simulink model "sgMdl_IO3xx_Resolver_Emulation_Setup"  (R2024b)
settings: Solver=FixedStepAuto  StartTime=0.0  StopTime=inf  RelTol=1e-3
undefined symbols (not defined in the file): Ended, Pull, pull, Single, up
libraries: speedgoatlib_fpga_analog_io x1, speedgoatlib_fpga_resolver x1, speedgoatlib_fpga x1
Description:
  | IO3xx Resolver Emulation - Setup
settings Model: ModifiedByFormat=Speedgoat  SimulationMode=external  ExtModeTrigDuration=100000  Creator=Speedgoat  LastModifiedBy=Speedgoat
settings SolverCC: ConcurrentTasks=on  PositivePriorityOrder=on
settings OptimizationCC: BlockReduction=off  OptimizeBlockIOStorage=off  ReuseModelBlockBuffer=off
settings DebuggingCC: TasksWithSamePriorityMsg=none
settings HardwareCC: ProdBitPerLong=64  ProdLongLongMode=on  ProdHWDeviceType=Intel->x86-64 (Linux 64)
settings ModelReferenceCC: EnableRefExpFcnMdlSchedulingChecks=on
settings RTWCC: Description=Speedgoat Real-Time Target Machine  SystemTargetFile=speedgoat.tlc  TemplateMakefile=slrealtime_default_tmf  Toolchain=Simulink Real-Time Toolchain  BuildConfiguration=Faster Runs  TargetLang=C++  GPUComputeCapability=3.5
settings SimulinkRealTimeTargetCC: SubcomponentCodeInterfacePackaging=Reusable function  InstructionSetFMA=off  LogToMDFFile=off  SLRTFileLogMaxRuns=10
settings ConfigComp: CovBoundaryAbsTol=1.0e-5

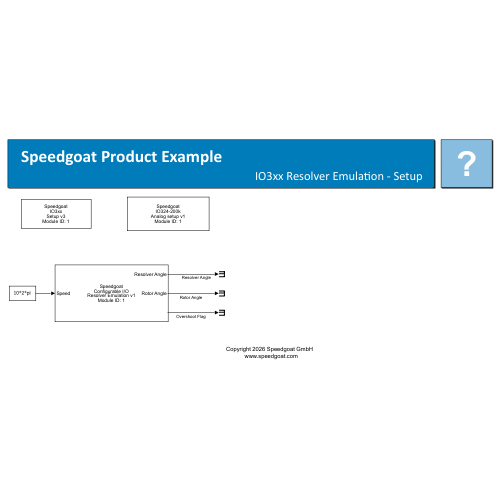
[thumbnail: Simulink's stored preview of the top-level diagram]
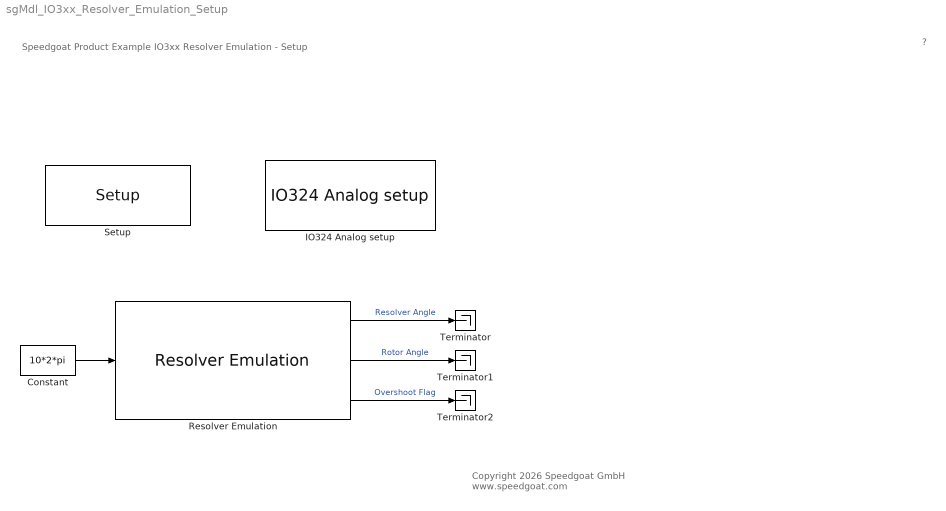
== system sgMdl_IO3xx_Resolver_Emulation_Setup ==
  note: Speedgoat Product Example
      | IO3xx Resolver Emulation - Setup
  note: ?
  note: Copyright 2026 Speedgoat GmbH
      |  www.speedgoat.com
  Constant : Constant  Value=10*2*pi  SampleTime=1e-3
  IO324 Analog setup : speedgoatlib_fpga_analog_io/IO324/IO324 Analog setup  id=1  parEnableCodeModule1=on  parEnableCodeModule2=off  parEnableCodeModule3=off  parEnableCodeModule4=off  parEnableCodeModule5=off  parEnableCodeModule6=off  parEnableCodeModule7=off  parEnableCodeModule8=off  parAdcEnableIndividualTrigger=off  parAdcTriggerMode1=I/O Module Internal Signal  parAdcSampleRate1=100e3  parAdcDioTriggerChannel1=1  parAdcInternalTrigger1=<empty>  parAdcOversampling1=None  parAdcTriggerMode2=Model Step  parAdcSampleRate2=100e3  parAdcDioTriggerChannel2=1  parAdcInternalTrigger2=<empty>  parAdcOversampling2=None  parAdcTriggerMode3=Model Step  parAdcSampleRate3=100e3  parAdcDioTriggerChannel3=1  parAdcInternalTrigger3=<empty>  parAdcOversampling3=None  parAdcTriggerMode4=Model Step  parAdcSampleRate4=100e3  parAdcDioTriggerChannel4=1  parAdcInternalTrigger4=<empty>  parAdcOversampling4=None  parAdcReadPrevValueIndividualTrigger=on  parAdcEnableFrame=off  parAdcTriggerMode=Model Step  parAdcReadPrevValue=off  parAdcSampleRate=100e3  parAdcDioTriggerChannel=1  parAdcInternalTrigger=<empty>  parAdcOversampling=None  parAdcTriggerResolution=1e-08  parAdcSampleRateFrame=100e3  parAdcFrameSize=-1  parAdcSampleTime=1e-3  parDacTriggerMode=I/O Module Internal Signal  parDacInternalTrigger=<empty>  parDacDioTriggerChannel=0  parDacEnableFrame=off  dacUsesTimer=off  parDacFifoThreshold=100  parDacTriggerResolution=1e-08  parDacSampleRate=5e6  parDacFrameSize=100  parDacSampleTime=-1  parAdcCoupling1=Single-Ended  parAdcChannel1=on  parAdcChannel2=off  parAdcChannel3=off  parAdcChannel4=off  parAdcChannel5=off  parAdcChannel6=off  parAdcChannel7=off  parAdcChannel8=off  parAdcRangeAll1=+-5.12 V  parVoltageRangePerChannelEn1=off  parAdcRange1=+-5.12 V  parAdcRange5=+-5.12 V  parAdcRange2=+-5.12 V  parAdcRange6=+-5.12 V  parAdcRange3=+-5.12 V  parAdcRange7=+-5.12 V  parAdcRange4=+-5.12 V  parAdcRange8=+-5.12 V  parAdcCoupling2=Single-Ended  parAdcChannel9=off  parAdcChannel10=off  parAdcChannel11=off  parAdcChannel12=off  parAdcChannel13=off  parAdcChannel14=off  parAdcChannel15=off  parAdcChannel16=off  parAdcRangeAll2=+-5.12 V  parVoltageRangePerChannelEn2=off  parAdcRange9=+-5.12 V  parAdcRange13=+-5.12 V  parAdcRange10=+-5.12 V  parAdcRange14=+-5.12 V  parAdcRange11=+-5.12 V  parAdcRange15=+-5.12 V  parAdcRange12=+-5.12 V  parAdcRange16=+-5.12 V  parAdcCoupling3=Single-Ended  parAdcChannel17=off  parAdcChannel18=off  parAdcChannel19=off  parAdcChannel20=off  parAdcChannel21=off  parAdcChannel22=off  parAdcChannel23=off  parAdcChannel24=off  parAdcRangeAll3=+-5.12 V  parVoltageRangePerChannelEn3=off  parAdcRange17=+-5.12 V  parAdcRange21=+-5.12 V  parAdcRange18=+-5.12 V  parAdcRange22=+-5.12 V  parAdcRange19=+-5.12 V  parAdcRange23=+-5.12 V  parAdcRange20=+-5.12 V  parAdcRange24=+-5.12 V  parAdcCoupling4=Single-Ended  parAdcChannel25=off  parAdcChannel26=off  parAdcChannel27=off  parAdcChannel28=off  parAdcChannel29=off  parAdcChannel30=off  parAdcChannel31=off  parAdcChannel32=off  parAdcRangeAll4=+-5.12 V  parVoltageRangePerChannelEn4=off  parAdcRange25=+-5.12 V  parAdcRange29=+-5.12 V  parAdcRange26=+-5.12 V  parAdcRange30=+-5.12 V  parAdcRange27=+-5.12 V  parAdcRange31=+-5.12 V  parAdcRange28=+-5.12 V  parAdcRange32=+-5.12 V  parAdcAutoCorrection=on  parDacChannel1=on  parDacChannel2=on  parDacChannel3=on  parDacChannel4=on  parDacChannel5=off  parDacChannel6=off  parDacChannel7=off  parDacChannel8=off  parDacRange1=+-5 V  parDacInitValue1=0  parDacReset1=on  parDacRange2=+-5 V  parDacInitValue2=0  parDacReset2=on  parDacRange3=+-5 V  parDacInitValue3=0  parDacReset3=on  parDacRange4=+-5 V  parDacInitValue4=0  parDacReset4=on  parDacRange5=+-5 V  parDacInitValue5=0  parDacReset5=on  parDacRange6=+-5 V  parDacInitValue6=0  parDacReset6=on  parDacRange7=+-5 V  parDacInitValue7=0  parDacReset7=on  parDacRange8=+-5 V  parDacInitValue8=0  parDacReset8=on  parDacAutoCorrection=on
      settings: SourceProductName=Analog IO
  Resolver Emulation : speedgoatlib_fpga_resolver/Resolver Emulation  id=1  chan=1  sampleTime=1e-3  tResolver=1e-6  board=Please select...  polePairs=1  angleOffset=0  selectSpeedPosition=Speed  initPosition=0  internExctSig=on  exctAmpl=5  exctFreq=1  exctOutEnable=off  gain=[1,1,1,1]  offset=[0,0,0,0]  phaseDelay=0  time_step_delay=0  showInExctFault=off  showInGain=off  showInOffset=off  showOutResAngle=on  showOutRotAngle=on  showOutOverFlag=on
      settings: SourceProductName=Resolver
  Setup : speedgoatlib_fpga/Setup/Setup  board=Please select...  id=1  pciSlot=-1  device_id=1  bitstreamFilePath=[]  bitstreamFile=Please select...  fpgaFreq=75e6  enableDma=off  rearEnb_1=off  rearIO_1=None  rearEnb_2=off  rearIO_2=None  ProgSpiFlash=off  ProgBPIFlash=off  useFpgaDmaController=off  dmaTrigDropdown=Model Step  dmaTrigSelect=0  dmaStopOnOverload=on  dmaModeSequential=on  dmaModeParallel=off  PullRPort15=pull-up 3.3V  PullRPort31=pull-up 3.3V  PullRPort47=pull-up 3.3V  PullRPort63=pull-up 3.3V  diffLineTermination_1=on  diffLineTermination_2=on  diffLineTermination_3=on  diffLineTermination_4=on  diffLineTermination_5=on  diffLineTermination_6=on  diffLineTermination_7=on  diffLineTermination_8=on  diffLineTermination_9=on  diffLineTermination_10=on  diffLineTermination_11=on  diffLineTermination_12=on  diffLineTermination_13=on  diffLineTermination_14=on  diffLineTermination_15=on  diffLineTermination_16=on  diffLineTermination_17=on  diffLineTermination_18=on  diffLineTermination_19=on  diffLineTermination_20=on  diffLineTermination_21=on  diffLineTermination_22=on  diffLineTermination_23=on  diffLineTermination_24=on  diffLineTermination_25=on  diffLineTermination_26=on  diffLineTermination_27=on  diffLineTermination_28=on  diffLineTermination_29=on  diffLineTermination_30=on  diffLineTermination_31=on  diffLineTermination_32=on  ioVoltageDropDown1=3.3V  pullResistorDropDown1_1=Pull-up  pullResistorDropDown1_2=Pull-up  pullResistorDropDown1_3=Pull-up  pullResistorDropDown1_4=Pull-up  pullResistorDropDown1_5=Pull-up  pullResistorDropDown1_6=Pull-up  pullResistorDropDown1_7=Pull-up  pullResistorDropDown1_8=Pull-up  ttlIsImplementedCheckBox1=off  pullResistorDropDown2=Pull-up  ioVoltageDropDown2=3.3V  ttlIsImplementedCheckBox2=off  pullResistorDropDown3=Pull-up  ioVoltageDropDown3=3.3V  ttlIsImplementedCheckBox3=off  pullResistorDropDown4=Pull-up  ioVoltageDropDown4=3.3V  ttlIsImplementedCheckBox4=off  pullResistorDropDown5=Pull-up  ioVoltageDropDown5=3.3V  ttlIsImplementedCheckBox5=off  pullResistorDropDown6=Pull-up  ioVoltageDropDown6=3.3V  ttlIsImplementedCheckBox6=off  pullResistorDropDown7=Pull-up  ioVoltageDropDown7=3.3V  ttlIsImplementedCheckBox7=off  pullResistorDropDown8=Pull-up  ioVoltageDropDown8=3.3V  ttlIsImplementedCheckBox8=off  terminationCheckBox1=off  terminationCheckBox2=off  terminationCheckBox3=off  terminationCheckBox4=off  diffIsImplementedCheckBox1=off  terminationCheckBox5=off  terminationCheckBox6=off  terminationCheckBox7=off  terminationCheckBox8=off  diffIsImplementedCheckBox2=off  terminationCheckBox9=off  terminationCheckBox10=off  terminationCheckBox11=off  terminationCheckBox12=off  diffIsImplementedCheckBox3=off  terminationCheckBox13=off  terminationCheckBox14=off  terminationCheckBox15=off  terminationCheckBox16=off  diffIsImplementedCheckBox4=off  terminationCheckBox17=off  terminationCheckBox18=off  terminationCheckBox19=off  terminationCheckBox20=off  diffIsImplementedCheckBox5=off  terminationCheckBox21=off  terminationCheckBox22=off  terminationCheckBox23=off  terminationCheckBox24=off  diffIsImplementedCheckBox6=off  terminationCheckBox25=off  terminationCheckBox26=off  terminationCheckBox27=off  terminationCheckBox28=off  diffIsImplementedCheckBox7=off  terminationCheckBox29=off  terminationCheckBox30=off  terminationCheckBox31=off  terminationCheckBox32=off  diffIsImplementedCheckBox8=off  PullRPort0_1=pull-up  VioPort0_1=3.3V  PullRPort1_1=pull-up  VioPort1_1=3.3V  PullRPort2_1=pull-up  VioPort2_1=3.3V  PullRPort3_1=pull-up  VioPort3_1=3.3V  PullRPort4_1=pull-up  VioPort4_1=3.3V  PullRPort5_1=pull-up  VioPort5_1=3.3V  PullRPort6_1=pull-up  VioPort6_1=3.3V  diffLineTermination_rear1_1=on  diffLineTermination_rear1_2=on  diffLineTermination_rear1_3=on  diffLineTermination_rear1_4=on  diffLineTermination_rear1_5=on  diffLineTermination_rear1_6=on  diffLineTermination_rear1_7=on  diffLineTermination_rear1_8=on  PullRPort0_2=pull-up  VioPort0_2=3.3V  PullRPort1_2=pull-up  VioPort1_2=3.3V  PullRPort2_2=pull-up  VioPort2_2=3.3V  PullRPort3_2=pull-up  VioPort3_2=3.3V  PullRPort4_2=pull-up  VioPort4_2=3.3V  PullRPort5_2=pull-up  VioPort5_2=3.3V  PullRPort6_2=pull-up  VioPort6_2=3.3V  diffLineTermination_rear2_1=on  diffLineTermination_rear2_2=on  diffLineTermination_rear2_3=on  diffLineTermination_rear2_4=on  diffLineTermination_rear2_5=on  diffLineTermination_rear2_6=on  diffLineTermination_rear2_7=on  diffLineTermination_rear2_8=on
      settings: SourceProductName=IO3xx
  Terminator : Terminator
  Terminator1 : Terminator
  Terminator2 : Terminator
  wires:
  Constant/1 -> Resolver Emulation/1
  Resolver Emulation/1 -> Terminator/1  "Resolver Angle"
  Resolver Emulation/2 -> Terminator1/1  "Rotor Angle"
  Resolver Emulation/3 -> Terminator2/1  "Overshoot Flag"
